simulink model "wrapper"  (R2025a)
settings: Solver=FixedStepDiscrete  StartTime=0.0  StopTime=10  FixedStep=SimulationStep  RelTol=1e-3
model workspace (MAT data in the model file):
  SimulationStep = Simulink.Parameter
  SimulationStep.Value = 0.01
  SimulationStep.Complexity = 'real'
  SimulationStep.Dimensions = [1 1]
  SimulationStep.DataType = 'auto'
settings Model: Creator=Gabriel Fernandes  LastModifiedBy=Gabriel Fernandes
settings OptimizationCC: UseDivisionForNetSlopeComputation=on  GainParamInheritBuiltInType=on  UseFloatMulNetSlope=on  OptimizeBlockIOStorage=off  BufferReuse=off  ReuseModelBlockBuffer=off  GlobalBufferReuse=off  ExpressionFolding=off  EnableMemcpy=off  PassReuseOutputArgsAs=Individual arguments  LocalBlockOutputs=off  ZeroExternalMemoryAtStartup=off  ZeroInternalMemoryAtStartup=off  NoFixptDivByZeroProtection=on  EfficientFloat2IntCast=on  LifeSpan=1  OptimizeDataStoreBuffers=off  BusAssignmentInplaceUpdate=off  OptimizationLevel=level0  OptimizationCustomize=off  EfficientTunableParamExpr=on
settings DebuggingCC: ParameterTunabilityLossMsg=error
settings HardwareCC: ProdLongLongMode=on
settings SFSimCC: MATLABDynamicMemAlloc=off
settings RTWCC: SystemTargetFile=ert.tlc  PackageGeneratedCodeAndArtifacts=on  PackageName=NoLinearBuild  TemplateMakefile=ert_default_tmf  BuildConfiguration=Debug  TargetLang=C++  Description=Embedded Coder
settings CodeAppCC: ForceParamTrailComments=on  IgnoreCustomStorageClasses=off  OperatorAnnotations=on  SimulinkDataObjDesc=on  SFDataObjDesc=on  CustomSymbolStrGlobalVar=rt$N$M  CustomSymbolStrType=$N$M  CustomSymbolStrFcn=$N$M$F  CustomSymbolStrMacro=$N$M  InsertBlockDesc=on
settings ERTTargetCC: ExtModeTransport=0.0  ExtModeStaticAlloc=off  ExtModeMexFile=ext_comm  ExtModeIntrfLevel=Level1  InlinedParameterPlacement=Hierarchical  RootIOFormat=Structure reference  ERTCustomFileTemplate=example_file_process.tlc  ERTFilePackagingFormat=CompactWithDataFile  TargetLangStandard=C++11 (ISO)  GenerateSampleERTMain=on  IncludeMdlTerminateFcn=off  CombineSignalStateStructs=on  SuppressErrorStatus=on  SupportAbsoluteTime=off  CodeInterfacePackaging=C++ class  SubcomponentCodeInterfacePackaging=C++ class  SupportComplex=off

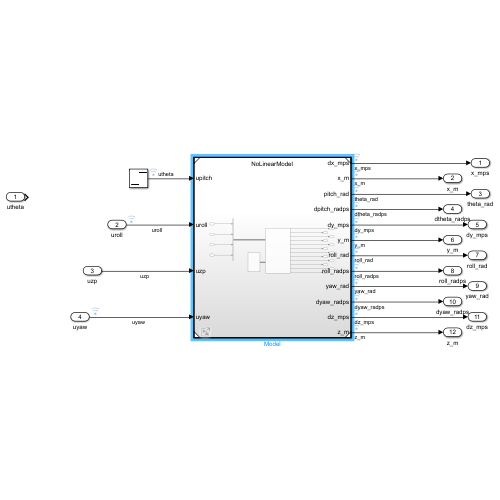
[thumbnail: Simulink's stored preview of the top-level diagram]
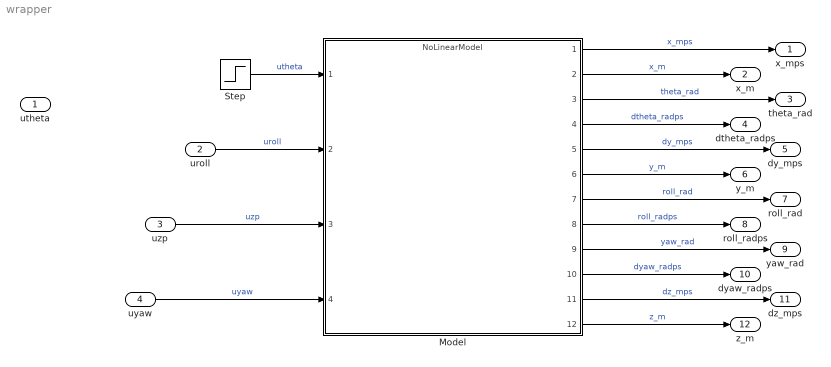
== system wrapper ==
  utheta : Inport
  uroll : Inport  Port=2
  uzp : Inport  Port=3
  uyaw : Inport  Port=4
  Model : ModelReference  ModelNameDialog=NoLinearModel.slx  UsingDefaultArgumentValue=0,0,0,0,0,0,0,0,0,0,0,0,0,0,0,0  SimulationMode=Normal  CodeInterface=Top model  ModelReferenceVersion=1.62
  Step : Step  SampleTime=0.01
  x_mps : Outport
  x_m : Outport  Port=2
  theta_rad : Outport  Port=3
  dtheta_radps : Outport  Port=4
  dy_mps : Outport  Port=5
  y_m : Outport  Port=6
  roll_rad : Outport  Port=7
  roll_radps : Outport  Port=8
  yaw_rad : Outport  Port=9
  dyaw_radps : Outport  Port=10
  dz_mps : Outport  Port=11
  z_m : Outport  Port=12
  wires:
  Step/1 -> Model/1  "utheta"
  Model/1 -> x_mps/1  "x_mps"
  Model/2 -> x_m/1  "x_m"
  Model/3 -> theta_rad/1  "theta_rad"
  Model/4 -> dtheta_radps/1  "dtheta_radps"
  uyaw/1 -> Model/4  "uyaw"
  uzp/1 -> Model/3  "uzp"
  uroll/1 -> Model/2  "uroll"
  Model/9 -> yaw_rad/1  "yaw_rad"
  Model/11 -> dz_mps/1  "dz_mps"
  Model/7 -> roll_rad/1  "roll_rad"
  Model/5 -> dy_mps/1  "dy_mps"
  Model/6 -> y_m/1  "y_m"
  Model/8 -> roll_radps/1  "roll_radps"
  Model/10 -> dyaw_radps/1  "dyaw_radps"
  Model/12 -> z_m/1  "z_m"
